simulink model "Final_Plant"  (R2024a)
settings: Solver=VariableStepAuto  StartTime=0.0  StopTime=inf  RelTol=1e-3
undefined symbols (not defined in the file): PropData
libraries: simulink x1
settings DataIOCC: SaveOutput=off  SaveTime=off

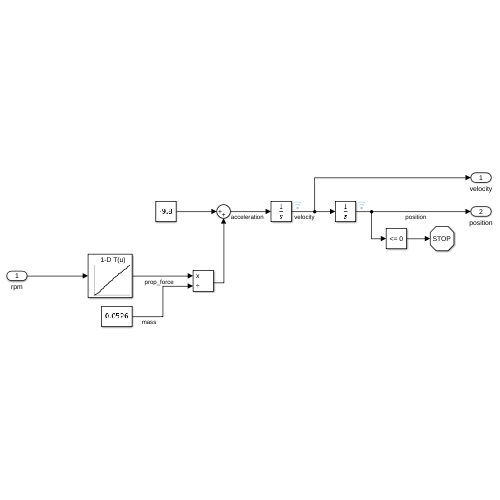
[thumbnail: Simulink's stored preview of the top-level diagram]
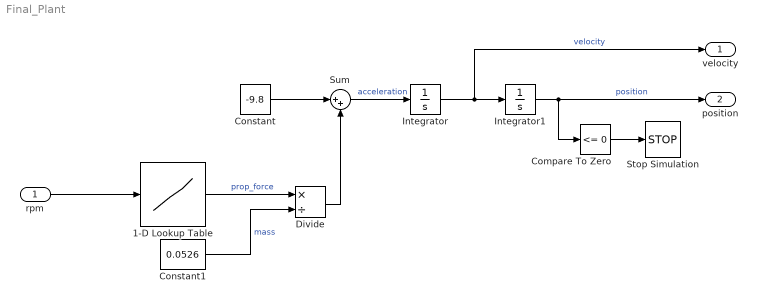
== system Final_Plant ==
  rpm : Inport  OutDataTypeStr=double  PortDimensions=1  SampleTime=[0,1]
  1-D Lookup Table : Lookup_n-D  NumberOfTableDimensions=1  BreakpointsForDimension1=PropData.rpm  Table=PropData.liftForce_N  InternalRulePriority=Speed  RndMeth=Simplest
  Compare To Zero : simulink/Logic and Bit Operations/Compare To Zero  relop=<=  OutDataTypeStr=boolean
  Constant : Constant  Value=-9.8
  Constant1 : Constant  Value=0.0526
  Divide : Product  Inputs=*/
  Integrator : Integrator  InitialCondition=0.5
  Integrator1 : Integrator  InitialCondition=2
  Stop Simulation : Stop
  Sum : Sum  Inputs=|++
  velocity : Outport  OutDataTypeStr=double  PortDimensions=1  SampleTime=0
  position : Outport  Port=2  OutDataTypeStr=double  PortDimensions=1  SampleTime=0
  wires:
  Constant1/1 -> Divide/2  "mass"
  Constant/1 -> Sum/1
  Divide/1 -> Sum/2
  rpm/1 -> 1-D Lookup Table/1
  Compare To Zero/1 -> Stop Simulation/1
  1-D Lookup Table/1 -> Divide/1  "prop_force"
  Integrator1/1 -> Compare To Zero/1, position/1  "position"
  Integrator/1 -> Integrator1/1, velocity/1  "velocity"
  Sum/1 -> Integrator/1  "acceleration"
